simulink model "pointOne_Simulink"  (R2022b)
settings: Solver=VariableStepAuto  StartTime=0.0  StopTime=010  MaxStep=1e-4  MinStep=1e-5  RelTol=1e-3
settings Model: Creator=yeyi5  LastModifiedBy=yeyi5

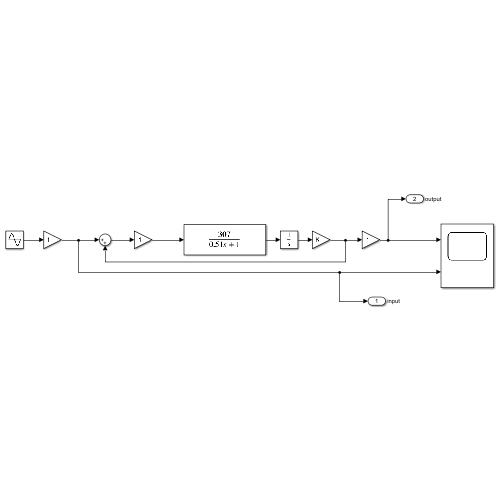
[thumbnail: Simulink's stored preview of the top-level diagram]
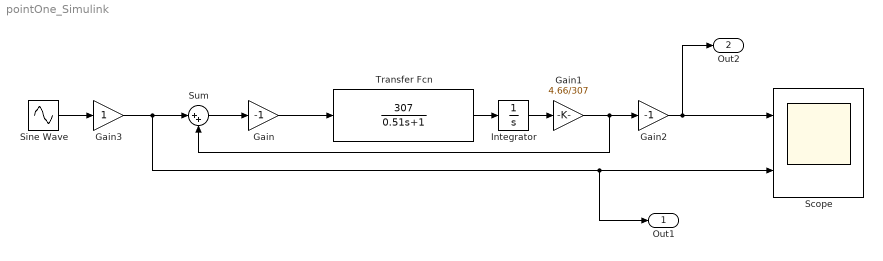
== system pointOne_Simulink ==
  Gain : Gain  Gain=-1
  Gain1 : Gain  Gain=4.66/307
  Gain2 : Gain  Gain=-1
  Gain3 : Gain
  Integrator : Integrator
  Scope : Scope  NumInputPorts=2
  Sine Wave : Sin  Amplitude=5  Frequency=1*(2 * pi)  SampleTime=0
  Sum : Sum  Inputs=|++
  Transfer Fcn : TransferFcn  Numerator=[307]  Denominator=[0.51 1]
  Out1 : Outport  SignalName=input
  Out2 : Outport  Port=2  SignalName=output
  wires:
  Transfer Fcn/1 -> Integrator/1
  Integrator/1 -> Gain1/1
  Gain2/1 -> Out2/1, Scope/1
  Sum/1 -> Gain/1
  Gain1/1 -> Sum/2, Gain2/1
  Sine Wave/1 -> Gain3/1
  Gain/1 -> Transfer Fcn/1
  Gain3/1 -> Out1/1, Scope/2, Sum/1
